simulink model "Sim_tanksmodel_FGS"  (R2020b)
settings: Solver=FixedStepAuto  StartTime=0.0  StopTime=7000  FixedStep=1  RelTol=1e-3  EnableMultiTasking=on
InitFcn:
  | cd ..
  | addpath(genpath('Algoritmo'))
  | cd ..
  | addpath(genpath('Sistema-Multitanque'))
  | cd FGS-PID\Simulacion
  | inParameters
undefined symbols (not defined in the file or in its folder): he1, he2, Kd1, Kd2, Kd3, Ki1, Ki2, Ki3, Kp1, Kp2, Kp3, Ts
libraries: simulink x2
settings Model: SimulationMode=accelerator  Creator=sahandar  LastModifiedBy=Usuario
settings SolverCC: AlgebraicLoopSolver=LineSearch
settings DataIOCC: LimitDataPoints=on  SaveFormat=Array  ReturnWorkspaceOutputs=off
settings OptimizationCC: LifeSpan=inf
settings DebuggingCC: AllowSymbolicDim=off  SFUnexpectedBacktrackingDiag=warning  SFNoUnconditionalDefaultTransitionDiag=warning  SFExecutionAtInitializationDiag=none  ArithmeticOperatorsInVariantConditions=warning
settings HardwareCC: ProdBitPerPointer=32  ProdBitPerSizeT=32  ProdBitPerPtrDiffT=32  ProdLargestAtomicFloat=None  ProdIntDivRoundTo=Undefined  ProdEndianess=Unspecified  ProdWordSize=32  ProdHWDeviceType=32-bit Generic
settings ModelReferenceCC: PropagateSignalLabelsOutOfModel=off
settings SFSimCC: SimUseLocalCustomCode=off  CustomCodeUndefinedFunction=UseInterfaceOnly
settings RTWCC: RTWUseLocalCustomCode=off
settings CodeAppCC: StateflowObjectComments=on
settings GRTTargetCC: TargetLangStandard=C89/C90 (ANSI)
settings ConfigComp: CovMetricSettings=dw  CovSaveCumulativeToWorkspaceVar=on  CovSaveSingleToWorkspaceVar=on  CovExternalEMLEnable=off

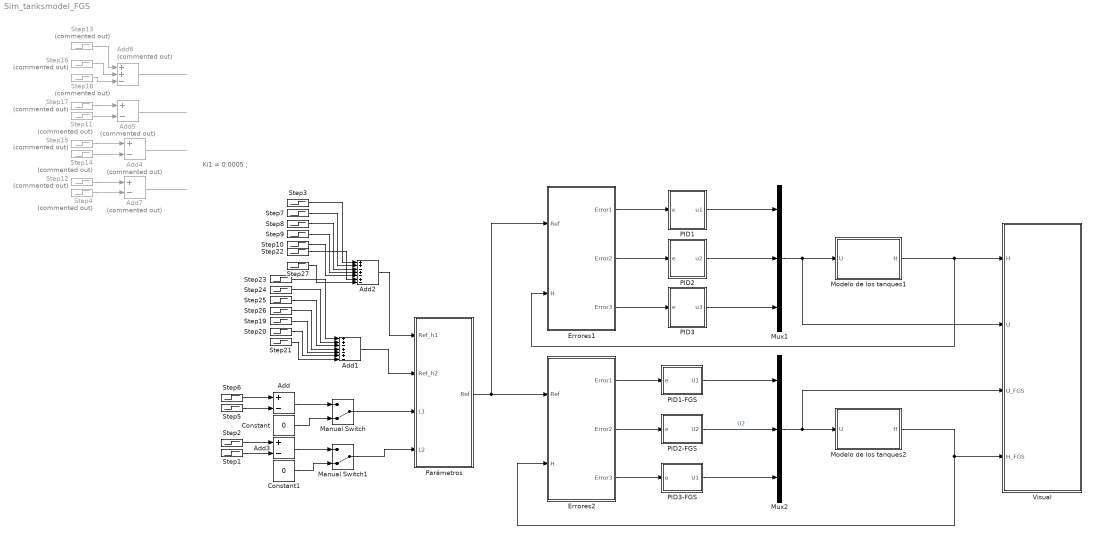
== system Sim_tanksmodel_FGS ==
  note: Ki1 = 0.0005 ;
  Add : Sum  Inputs=+-
  Add1 : Sum  Inputs=++-+-+-
  Add2 : Sum  Inputs=++-+-+-
  Add3 : Sum  Inputs=+-
  Add4 : Sum  Commented=on  Inputs=+-
  Add5 : Sum  Commented=on  Inputs=+-
  Add6 : Sum  Commented=on  Inputs=++-
  Add7 : Sum  Commented=on  Inputs=+-
  Constant : Constant  Value=0
  Constant1 : Constant  Value=0
  Errores1 : Subsystem
  Errores2 : Subsystem
  Manual Switch : ManualSwitch  CurrentSetting=0
  Manual Switch1 : ManualSwitch  CurrentSetting=0
  Modelo de los tanques1 : Subsystem
  Modelo de los tanques2 : Subsystem
  Mux1 : Mux  Inputs=3
  Mux2 : Mux  Inputs=3
  PID1 : Subsystem
  PID1-FGS : Subsystem
  PID2 : Subsystem
  PID2-FGS : Subsystem
  PID3 : Subsystem
  PID3-FGS : Subsystem
  Parámetros : Subsystem
  Step1 : Step  Time=1900  SampleTime=Ts
  Step10 : Step  Time=4000  After=0.06  SampleTime=Ts
  Step11 : Step  Commented=on  Time=900  After=0.03  SampleTime=Ts
  Step12 : Step  Commented=on  Time=1850  SampleTime=Ts
  Step13 : Step  Commented=on  Time=10  Before=he1  After=0.10  SampleTime=Ts
  Step14 : Step  Commented=on  Time=1800  SampleTime=Ts
  Step15 : Step  Commented=on  Time=1600  SampleTime=Ts
  Step16 : Step  Commented=on  Time=10  Before=he1  After=0.10  SampleTime=Ts
  Step17 : Step  Commented=on  Time=10  Before=he2  After=0.07  SampleTime=Ts
  Step18 : Step  Commented=on  Time=900  After=0.05  SampleTime=Ts
  Step19 : Step  Time=4000  After=0.06  SampleTime=Ts
  Step2 : Step  Time=1850  SampleTime=Ts
  Step20 : Step  Time=5000  After=0.06  SampleTime=Ts
  Step21 : Step  Time=6000  After=0.06  SampleTime=Ts
  Step22 : Step  Time=5000  After=0.06  SampleTime=Ts
  Step23 : Step  Time=0  Before=he1  After=0.02  SampleTime=Ts
  Step24 : Step  Time=1000  After=0.06  SampleTime=Ts
  Step25 : Step  Time=1500  After=0.06  SampleTime=Ts
  Step26 : Step  Time=3000  After=0.06  SampleTime=Ts
  Step27 : Step  Time=6000  After=0.06  SampleTime=Ts
  Step3 : Step  Time=0  Before=he1  After=0.02  SampleTime=Ts
  Step4 : Step  Commented=on  Time=1900  SampleTime=Ts
  Step5 : Step  Time=1800  SampleTime=Ts
  Step6 : Step  Time=1600  SampleTime=Ts
  Step7 : Step  Time=1000  After=0.06  SampleTime=Ts
  Step8 : Step  Time=1500  After=0.06  SampleTime=Ts
  Step9 : Step  Time=3000  After=0.06  SampleTime=Ts
  Visual : Subsystem
  wires:
  Mux1/1 -> Visual/2(U), Modelo de los tanques1/1(U)
  Step6/1 -> Add/1
  Step5/1 -> Add/2
  Modelo de los tanques1/1(H) -> Errores1/2(H), Visual/1(H)
  Step7/1 -> Add2/2
  Step1/1 -> Add3/2
  Step2/1 -> Add3/1
  PID3-FGS/1(U1) -> Mux2/3
  Errores2/3(Error3) -> PID3-FGS/1(e)
  PID2-FGS/1(U2) -> Mux2/2  "U2"
  Errores2/2(Error2) -> PID2-FGS/1(e)
  PID1-FGS/1(U1) -> Mux2/1
  Errores2/1(Error1) -> PID1-FGS/1(e)
  Modelo de los tanques2/1(H) -> Errores2/2(H), Visual/4(H_FGS)
  Parámetros/1(Ref) -> Errores2/1(Ref), Errores1/1(Ref)
  Mux2/1 -> Visual/3(U_FGS), Modelo de los tanques2/1(U)
  PID2/1(u2) -> Mux1/2
  PID3/1(u3) -> Mux1/3
  Errores1/2(Error2) -> PID2/1(e)
  Errores1/3(Error3) -> PID3/1(e)
  Errores1/1(Error1) -> PID1/1(e)
  PID1/1(u1) -> Mux1/1
  Step9/1 -> Add2/4
  Add2/1 -> Parámetros/1(Ref_h1)
  Step3/1 -> Add2/1
  Step13/1 -> Add6/1
  Add4/1 -> ?
  Step16/1 -> Add6/2
  Step17/1 -> Add5/1
  Add7/1 -> ?
  Add5/1 -> ?
  Step4/1 -> Add7/2
  Add6/1 -> ?
  Step12/1 -> Add7/1
  Step15/1 -> Add4/1
  Step14/1 -> Add4/2
  Step11/1 -> Add5/2
  Step18/1 -> Add6/3
  Add/1 -> Manual Switch/1
  Manual Switch/1 -> Parámetros/3(L1)
  Add3/1 -> Manual Switch1/1
  Manual Switch1/1 -> Parámetros/4(L2)
  Constant/1 -> Manual Switch/2
  Constant1/1 -> Manual Switch1/2
  Step8/1 -> Add2/3
  Step10/1 -> Add2/5
  Step22/1 -> Add2/6
  Add1/1 -> Parámetros/2(Ref_h2)
  Step27/1 -> Add2/7
  Step21/1 -> Add1/7
  Step20/1 -> Add1/6
  Step19/1 -> Add1/5
  Step25/1 -> Add1/3
  Step23/1 -> Add1/1
  Step26/1 -> Add1/4
  Step24/1 -> Add1/2

== system Sim_tanksmodel_FGS/Errores1 ==
  Ref : Inport
  H : Inport  Port=2
  Add : Sum  Inputs=+-
  Add1 : Sum  Inputs=+-
  Add4 : Sum  Inputs=-+
  Demux : Demux  Outputs=2
  Demux1 : Demux  Outputs=2
  Error1 : Outport
  Error2 : Outport  Port=2
  Error3 : Outport  Port=3
  wires:
  Ref/1 -> Demux/1
  Demux1/2 -> Add1/2  "h2"
  Demux1/1 -> Add/2  "h1"
  Demux/2 -> Add1/1  "ref_h2"
  H/1 -> Demux1/1
  Demux/1 -> Add/1  "ref_h1"
  Add/1 -> Add4/1, Error1/1
  Add1/1 -> Add4/2, Error3/1
  Add4/1 -> Error2/1

== system Sim_tanksmodel_FGS/Errores2 ==
  Ref : Inport
  H : Inport  Port=2
  Add : Sum  Inputs=+-
  Add1 : Sum  Inputs=+-
  Add4 : Sum  Inputs=-+
  Demux : Demux  Outputs=2
  Demux1 : Demux  Outputs=2
  Error1 : Outport
  Error2 : Outport  Port=2
  Error3 : Outport  Port=3
  wires:
  Demux1/2 -> Add1/2  "h2"
  Demux1/1 -> Add/2  "h1"
  Ref/1 -> Demux/1
  Demux/1 -> Add/1  "ref_h1"
  Add1/1 -> Add4/2, Error3/1
  Add4/1 -> Error2/1
  H/1 -> Demux1/1
  Add/1 -> Add4/1, Error1/1
  Demux/2 -> Add1/1  "ref_h2"

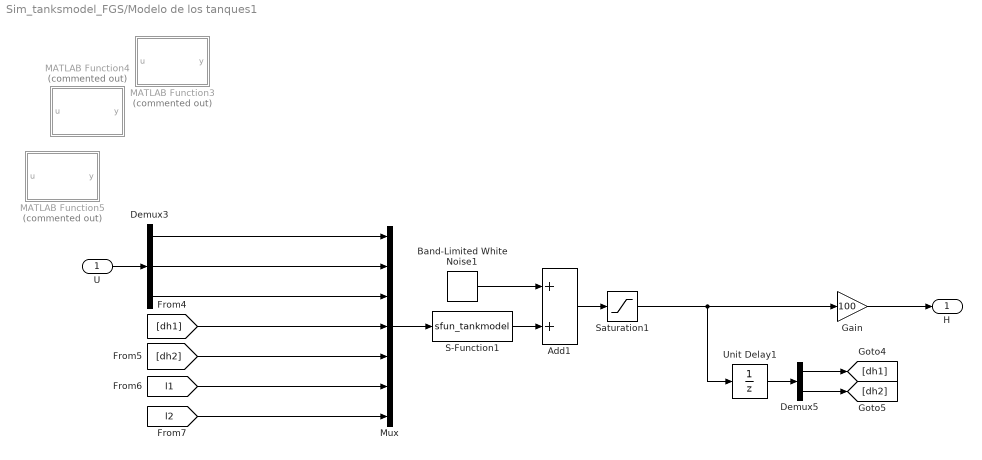
== system Sim_tanksmodel_FGS/Modelo de los tanques1 ==
  U : Inport
  Add1 : Sum
  Band-Limited White Noise1 : simulink/Sources/Band-Limited White Noise  Cov=N  Ts=Ts  seed=[23341]
  Demux3 : Demux  Outputs=3
  Demux5 : Demux  Outputs=2
  Gain : Gain  Gain=100
  MATLAB Function3 : MATLAB Function  Commented=on  TreatAsAtomicUnit=on
  MATLAB Function4 : MATLAB Function  Commented=on  TreatAsAtomicUnit=on
  MATLAB Function5 : MATLAB Function  Commented=on  TreatAsAtomicUnit=on
  Mux : Mux  Inputs=7
  S-Function1 : S-Function  FunctionName=sfun_tankmodel  Parameters=vars  SFunctionDeploymentMode=off  EnableBusSupport=off
  Saturation1 : Saturate  UpperLimit=inf  LowerLimit=0
  Unit Delay1 : UnitDelay  SampleTime=-1  HasFrameUpgradeWarning=on
  H : Outport  VectorParamsAs1DForOutWhenUnconnected=off
  wires:
  Saturation1/1 -> Unit Delay1/1, Gain/1
  Band-Limited White Noise1/1 -> Add1/1
  [l2] -> Mux/7
  [l1] -> Mux/6
  S-Function1/1 -> Add1/2
  [dh2] -> Mux/5
  Add1/1 -> Saturation1/1
  U/1 -> Demux3/1
  [dh1] -> Mux/4
  Mux/1 -> S-Function1/1
  Unit Delay1/1 -> Demux5/1
  Demux5/1 -> [dh1]
  Demux5/2 -> [dh2]
  Gain/1 -> H/1
  Demux3/1 -> Mux/1
  Demux3/2 -> Mux/2
  Demux3/3 -> Mux/3

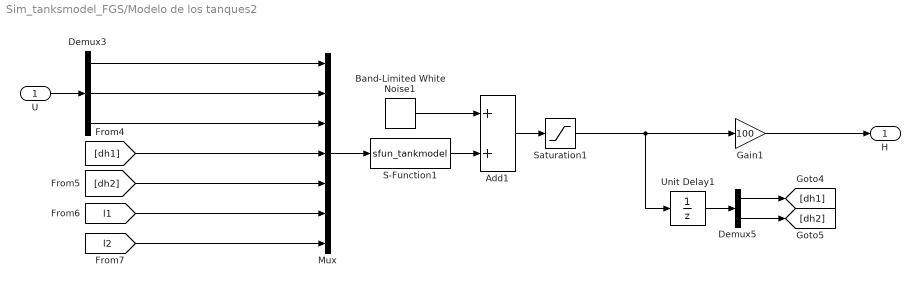
== system Sim_tanksmodel_FGS/Modelo de los tanques2 ==
  U : Inport
  Add1 : Sum
  Band-Limited White Noise1 : simulink/Sources/Band-Limited White Noise  Cov=N  Ts=Ts  seed=[23341]
  Demux3 : Demux  Outputs=3
  Demux5 : Demux  Outputs=2
  Gain1 : Gain  Gain=100
  Mux : Mux  Inputs=7
  S-Function1 : S-Function  FunctionName=sfun_tankmodel  Parameters=vars  SFunctionDeploymentMode=off  EnableBusSupport=off
  Saturation1 : Saturate  UpperLimit=inf  LowerLimit=0
  Unit Delay1 : UnitDelay  SampleTime=-1  HasFrameUpgradeWarning=on
  H : Outport  VectorParamsAs1DForOutWhenUnconnected=off
  wires:
  Demux5/2 -> [dh2]
  Demux5/1 -> [dh1]
  Unit Delay1/1 -> Demux5/1
  Mux/1 -> S-Function1/1
  [dh1] -> Mux/4
  Demux3/1 -> Mux/1
  U/1 -> Demux3/1
  Add1/1 -> Saturation1/1
  Demux3/3 -> Mux/3
  [dh2] -> Mux/5
  S-Function1/1 -> Add1/2
  [l1] -> Mux/6
  [l2] -> Mux/7
  Band-Limited White Noise1/1 -> Add1/1
  Demux3/2 -> Mux/2
  Saturation1/1 -> Gain1/1, Unit Delay1/1
  Gain1/1 -> H/1

== system Sim_tanksmodel_FGS/PID1 ==
  e : Inport
  Constant : Constant  Value=Kp1
  Constant1 : Constant  Value=Ki1
  Constant2 : Constant  Value=Kd1
  PID Controller : Subsystem
  Saturation : Saturate  UpperLimit=1  LowerLimit=0
  u1 : Outport
  wires:
  Constant2/1 -> PID Controller/4(Kd)
  Constant1/1 -> PID Controller/3(Ki)
  Constant/1 -> PID Controller/2(Kp)
  e/1 -> PID Controller/1(e)
  PID Controller/1(u) -> Saturation/1
  Saturation/1 -> u1/1

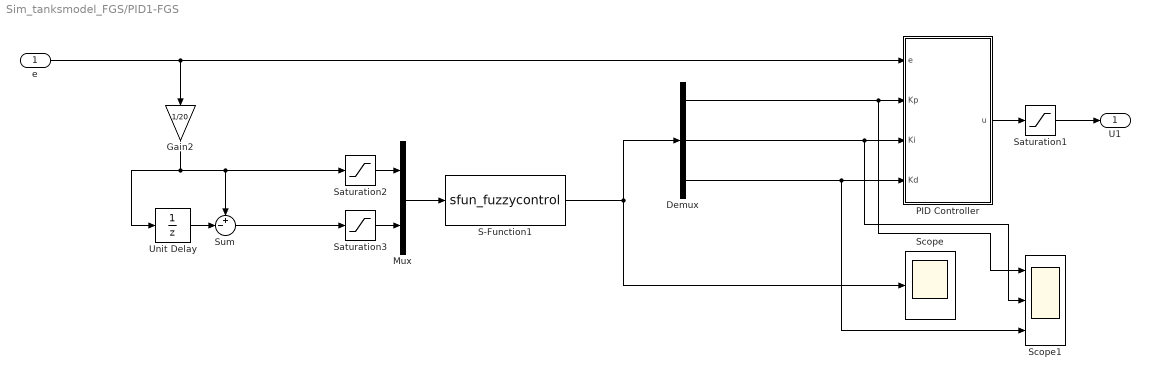
== system Sim_tanksmodel_FGS/PID1-FGS ==
  e : Inport
  Demux : Demux  Outputs=3
  Gain2 : Gain  Gain=1/20
  Mux : Mux  Inputs=2
  PID Controller : Subsystem
  S-Function1 : S-Function  FunctionName=sfun_fuzzycontrol  Parameters=range_gains1  SFunctionDeploymentMode=off  EnableBusSupport=off
  Saturation1 : Saturate  UpperLimit=1  LowerLimit=0
  Saturation2 : Saturate  UpperLimit=1  LowerLimit=-1
  Saturation3 : Saturate  UpperLimit=1  LowerLimit=-1
  Scope : Scope
  Scope1 : Scope  NumInputPorts=3
  Sum : Sum  Inputs=+-|
  Unit Delay : UnitDelay  SampleTime=-1
  U1 : Outport
  wires:
  Unit Delay/1 -> Sum/2
  Mux/1 -> S-Function1/1
  S-Function1/1 -> Demux/1, Scope/1
  Saturation1/1 -> U1/1
  Demux/1 -> Scope1/1, PID Controller/2(Kp)
  Demux/3 -> Scope1/3, PID Controller/4(Kd)
  PID Controller/1(u) -> Saturation1/1
  Demux/2 -> Scope1/2, PID Controller/3(Ki)
  Saturation2/1 -> Mux/1
  Saturation3/1 -> Mux/2
  e/1 -> Gain2/1, PID Controller/1(e)
  Sum/1 -> Saturation3/1
  Gain2/1 -> Unit Delay/1, Saturation2/1, Sum/1

== system Sim_tanksmodel_FGS/PID2 ==
  e : Inport
  Constant : Constant  Value=Kp2
  Constant1 : Constant  Value=Ki2
  Constant2 : Constant  Value=Kd2
  PID Controller : Subsystem
  Saturation : Saturate  UpperLimit=1  LowerLimit=0
  u2 : Outport
  wires:
  Saturation/1 -> u2/1
  e/1 -> PID Controller/1(e)
  Constant/1 -> PID Controller/2(Kp)
  Constant1/1 -> PID Controller/3(Ki)
  Constant2/1 -> PID Controller/4(Kd)
  PID Controller/1(u) -> Saturation/1

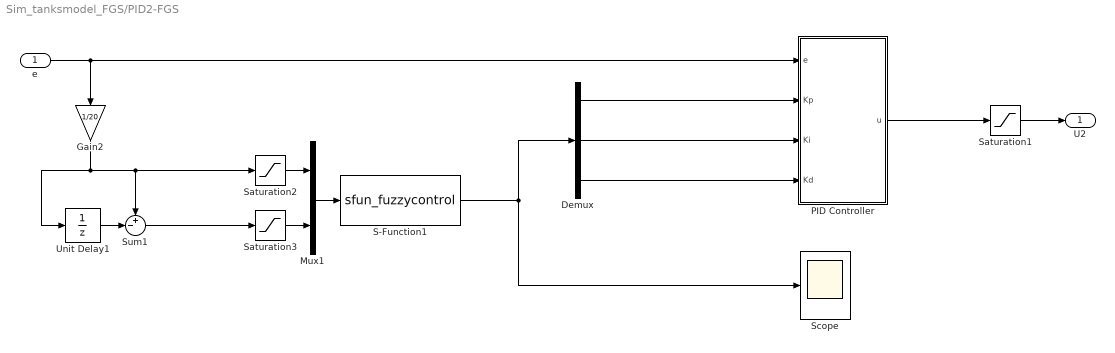
== system Sim_tanksmodel_FGS/PID2-FGS ==
  e : Inport
  Demux : Demux  Outputs=3
  Gain2 : Gain  Gain=1/20
  Mux1 : Mux  Inputs=2
  PID Controller : Subsystem
  S-Function1 : S-Function  FunctionName=sfun_fuzzycontrol  Parameters=range_gains2  SFunctionDeploymentMode=off  EnableBusSupport=off
  Saturation1 : Saturate  UpperLimit=1  LowerLimit=0
  Saturation2 : Saturate  UpperLimit=1  LowerLimit=-1
  Saturation3 : Saturate  UpperLimit=1  LowerLimit=-1
  Scope : Scope
  Sum1 : Sum  Inputs=+-|
  Unit Delay1 : UnitDelay  SampleTime=-1
  U2 : Outport
  wires:
  Demux/2 -> PID Controller/3(Ki)
  Demux/1 -> PID Controller/2(Kp)
  Demux/3 -> PID Controller/4(Kd)
  Saturation1/1 -> U2/1
  S-Function1/1 -> Demux/1, Scope/1
  PID Controller/1(u) -> Saturation1/1
  Unit Delay1/1 -> Sum1/2
  Mux1/1 -> S-Function1/1
  Saturation3/1 -> Mux1/2
  Saturation2/1 -> Mux1/1
  e/1 -> PID Controller/1(e), Gain2/1
  Sum1/1 -> Saturation3/1
  Gain2/1 -> Unit Delay1/1, Saturation2/1, Sum1/1

== system Sim_tanksmodel_FGS/PID3 ==
  e : Inport
  Constant : Constant  Value=Kp3
  Constant1 : Constant  Value=Ki3
  Constant2 : Constant  Value=Kd3
  Gain : Gain  Gain=-1
  PID Controller : Subsystem
  Saturation : Saturate  UpperLimit=1  LowerLimit=0
  u3 : Outport
  wires:
  Constant2/1 -> PID Controller/4(Kd)
  Constant1/1 -> PID Controller/3(Ki)
  Constant/1 -> PID Controller/2(Kp)
  e/1 -> PID Controller/1(e)
  Saturation/1 -> u3/1
  PID Controller/1(u) -> Gain/1
  Gain/1 -> Saturation/1

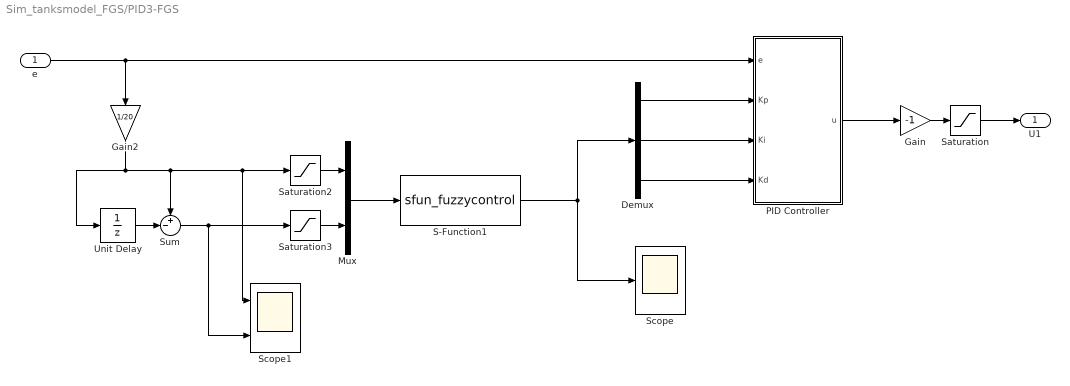
== system Sim_tanksmodel_FGS/PID3-FGS ==
  e : Inport
  Demux : Demux  Outputs=3
  Gain : Gain  Gain=-1
  Gain2 : Gain  Gain=1/20
  Mux : Mux  Inputs=2
  PID Controller : Subsystem
  S-Function1 : S-Function  FunctionName=sfun_fuzzycontrol  Parameters=range_gains3  SFunctionDeploymentMode=off  EnableBusSupport=off
  Saturation : Saturate  UpperLimit=1  LowerLimit=0
  Saturation2 : Saturate  UpperLimit=1  LowerLimit=-1
  Saturation3 : Saturate  UpperLimit=1  LowerLimit=-1
  Scope : Scope
  Scope1 : Scope  NumInputPorts=2
  Sum : Sum  Inputs=+-|
  Unit Delay : UnitDelay  SampleTime=-1
  U1 : Outport
  wires:
  Demux/2 -> PID Controller/3(Ki)
  Demux/1 -> PID Controller/2(Kp)
  Demux/3 -> PID Controller/4(Kd)
  Saturation/1 -> U1/1
  S-Function1/1 -> Demux/1, Scope/1
  Gain/1 -> Saturation/1
  PID Controller/1(u) -> Gain/1
  Unit Delay/1 -> Sum/2
  Mux/1 -> S-Function1/1
  Saturation3/1 -> Mux/2
  Saturation2/1 -> Mux/1
  e/1 -> PID Controller/1(e), Gain2/1
  Sum/1 -> Scope1/2, Saturation3/1
  Gain2/1 -> Unit Delay/1, Scope1/1, Saturation2/1, Sum/1

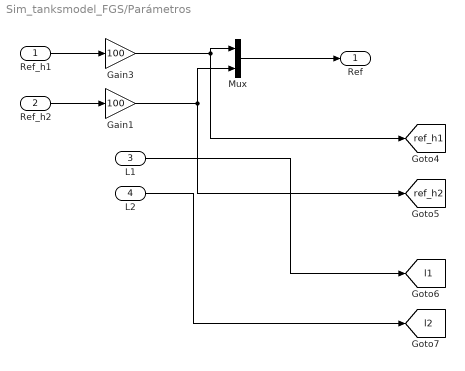
== system Sim_tanksmodel_FGS/Parámetros ==
  Ref_h1 : Inport
  Ref_h2 : Inport  Port=2
  L1 : Inport  Port=3
  L2 : Inport  Port=4
  Gain1 : Gain  Gain=100
  Gain3 : Gain  Gain=100
  Mux : Mux  Inputs=2
  Ref : Outport
  tag scope: l1=global, l2=global, ref_h1=global, ref_h2=global
  wires:
  L1/1 -> [l1]
  Mux/1 -> Ref/1
  Ref_h1/1 -> Gain3/1
  L2/1 -> [l2]
  Ref_h2/1 -> Gain1/1
  Gain3/1 -> Mux/1, [ref_h1]
  Gain1/1 -> [ref_h2], Mux/2

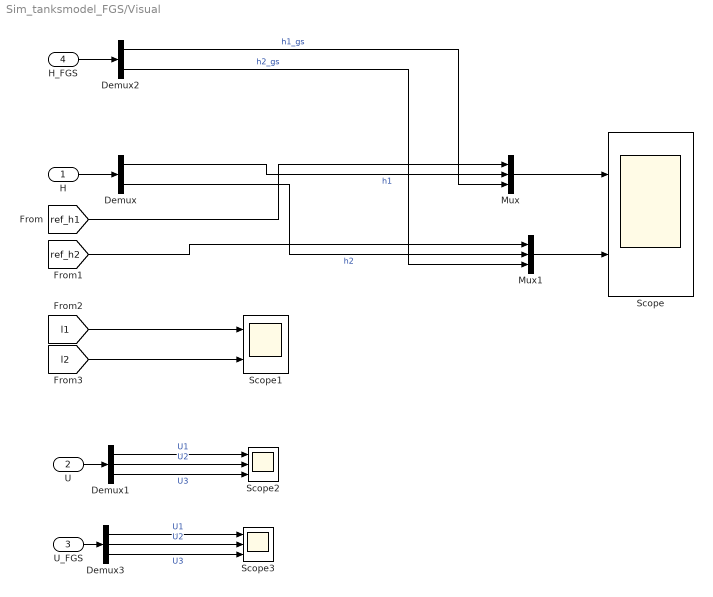
== system Sim_tanksmodel_FGS/Visual ==
  H : Inport
  U : Inport  Port=2
  U_FGS : Inport  Port=3
  H_FGS : Inport  Port=4
  Demux : Demux  Outputs=2
  Demux1 : Demux  Outputs=3
  Demux2 : Demux  Outputs=2
  Demux3 : Demux  Outputs=3
  Mux : Mux  Inputs=3
  Mux1 : Mux  Inputs=3
  Scope : Scope  NumInputPorts=2
  Scope1 : Scope  NumInputPorts=2
  Scope2 : Scope  NumInputPorts=3
  Scope3 : Scope  NumInputPorts=3
  wires:
  H/1 -> Demux/1
  Demux/1 -> Mux/2  "h1"
  [ref_h1] -> Mux/1
  Mux/1 -> Scope/1
  Demux/2 -> Mux1/2  "h2"
  [ref_h2] -> Mux1/1
  [l1] -> Scope1/1
  [l2] -> Scope1/2
  U/1 -> Demux1/1
  Demux1/1 -> Scope2/1  "U1"
  Demux1/2 -> Scope2/2  "U2"
  Demux1/3 -> Scope2/3  "U3"
  Mux1/1 -> Scope/2
  Demux2/1 -> Mux/3  "h1_gs"
  H_FGS/1 -> Demux2/1
  Demux2/2 -> Mux1/3  "h2_gs"
  Demux3/3 -> Scope3/3  "U3"
  Demux3/2 -> Scope3/2  "U2"
  Demux3/1 -> Scope3/1  "U1"
  U_FGS/1 -> Demux3/1

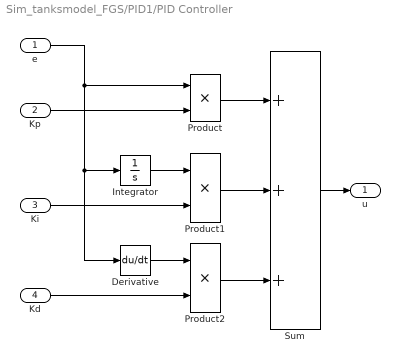
== system Sim_tanksmodel_FGS/PID1/PID Controller ==
  e : Inport
  Kp : Inport  Port=2
  Ki : Inport  Port=3
  Kd : Inport  Port=4
  Derivative : Derivative
  Integrator : Integrator
  Product : Product
  Product1 : Product
  Product2 : Product
  Sum : Sum  Inputs=3
  u : Outport
  wires:
  Sum/1 -> u/1
  Product/1 -> Sum/1
  Kp/1 -> Product/2
  Ki/1 -> Product1/2
  Integrator/1 -> Product1/1
  Product1/1 -> Sum/2
  Product2/1 -> Sum/3
  Kd/1 -> Product2/2
  e/1 -> Derivative/1, Integrator/1, Product/1
  Derivative/1 -> Product2/1

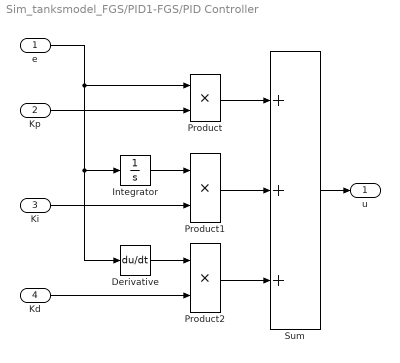
== system Sim_tanksmodel_FGS/PID1-FGS/PID Controller ==
  e : Inport
  Kp : Inport  Port=2
  Ki : Inport  Port=3
  Kd : Inport  Port=4
  Derivative : Derivative
  Integrator : Integrator
  Product : Product
  Product1 : Product
  Product2 : Product
  Sum : Sum  Inputs=3
  u : Outport
  wires:
  Sum/1 -> u/1
  Product/1 -> Sum/1
  Kp/1 -> Product/2
  Ki/1 -> Product1/2
  Integrator/1 -> Product1/1
  Product1/1 -> Sum/2
  Product2/1 -> Sum/3
  Kd/1 -> Product2/2
  e/1 -> Derivative/1, Integrator/1, Product/1
  Derivative/1 -> Product2/1

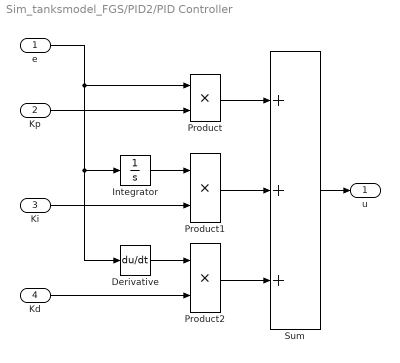
== system Sim_tanksmodel_FGS/PID2/PID Controller ==
  e : Inport
  Kp : Inport  Port=2
  Ki : Inport  Port=3
  Kd : Inport  Port=4
  Derivative : Derivative
  Integrator : Integrator
  Product : Product
  Product1 : Product
  Product2 : Product
  Sum : Sum  Inputs=3
  u : Outport
  wires:
  Derivative/1 -> Product2/1
  e/1 -> Product/1, Integrator/1, Derivative/1
  Kd/1 -> Product2/2
  Product2/1 -> Sum/3
  Product1/1 -> Sum/2
  Integrator/1 -> Product1/1
  Ki/1 -> Product1/2
  Kp/1 -> Product/2
  Product/1 -> Sum/1
  Sum/1 -> u/1

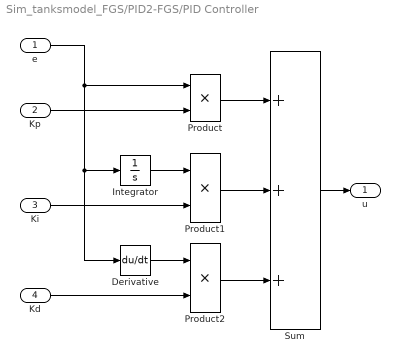
== system Sim_tanksmodel_FGS/PID2-FGS/PID Controller ==
  e : Inport
  Kp : Inport  Port=2
  Ki : Inport  Port=3
  Kd : Inport  Port=4
  Derivative : Derivative
  Integrator : Integrator
  Product : Product
  Product1 : Product
  Product2 : Product
  Sum : Sum  Inputs=3
  u : Outport
  wires:
  Sum/1 -> u/1
  Product/1 -> Sum/1
  Kp/1 -> Product/2
  Ki/1 -> Product1/2
  Integrator/1 -> Product1/1
  Product1/1 -> Sum/2
  Product2/1 -> Sum/3
  Kd/1 -> Product2/2
  e/1 -> Derivative/1, Integrator/1, Product/1
  Derivative/1 -> Product2/1

== system Sim_tanksmodel_FGS/PID3/PID Controller ==
  e : Inport
  Kp : Inport  Port=2
  Ki : Inport  Port=3
  Kd : Inport  Port=4
  Derivative : Derivative
  Integrator : Integrator
  Product : Product
  Product1 : Product
  Product2 : Product
  Sum : Sum  Inputs=3
  u : Outport
  wires:
  Sum/1 -> u/1
  Product/1 -> Sum/1
  Kp/1 -> Product/2
  Ki/1 -> Product1/2
  Integrator/1 -> Product1/1
  Product1/1 -> Sum/2
  Product2/1 -> Sum/3
  Kd/1 -> Product2/2
  e/1 -> Derivative/1, Integrator/1, Product/1
  Derivative/1 -> Product2/1

== system Sim_tanksmodel_FGS/PID3-FGS/PID Controller ==
  e : Inport
  Kp : Inport  Port=2
  Ki : Inport  Port=3
  Kd : Inport  Port=4
  Derivative : Derivative
  Integrator : Integrator
  Product : Product
  Product1 : Product
  Product2 : Product
  Sum : Sum  Inputs=3
  u : Outport
  wires:
  Sum/1 -> u/1
  Product/1 -> Sum/1
  Kp/1 -> Product/2
  Ki/1 -> Product1/2
  Integrator/1 -> Product1/1
  Product1/1 -> Sum/2
  Product2/1 -> Sum/3
  Kd/1 -> Product2/2
  e/1 -> Derivative/1, Integrator/1, Product/1
  Derivative/1 -> Product2/1

== matlab function Sim_tanksmodel_FGS/Modelo de los tanques1/MATLAB Function4 ==
  data: u input; y output
function y = fcn(u)
y =  2.189*u^5 - 5.942*u^4 + 6.022*u^3 - 2.835*u^2 + 0.7665*u + 0.0489;

== matlab function Sim_tanksmodel_FGS/Modelo de los tanques1/MATLAB Function5 ==
  data: u input; y output
function y = fcn(u)
y =  12.35*u^5 - 28.71*u^4 + 25.11*u^3 - 9.510*u^2 + 1.609*u + 0.09998;

== matlab function Sim_tanksmodel_FGS/Modelo de los tanques1/MATLAB Function3 ==
  data: u input; y output
function y = fcn(u)
y = u
if   0 <= u && u <= 0.0253
  y = (9.578 * 10^5 * (u)^(4.45)) + 0.05;
end
if   0.0253 < u && u <= 0.2342
  y =  -0.08032*(u)^(-0.1767) + 0.2788;
end
    
if   0.2342 < u && u <= 1
 y = 0.1647*exp(0.3041*u) + 2.551*10^(-17)*exp(34.57*u);
end
